simulink model "testRadiationDivisionInclined"  (R2018b)
settings: Solver=ode45  StartTime=0.0  StopTime=365*24*3600  MaxStep=100  RelTol=1e-3  EnableMultiTasking=on
undefined symbols (not defined in the file): Germany, path_carnot, Potsdam
libraries: carnot x3, Radiation_Divison x1
settings Model: Creator=drhf  LastModifiedBy=drhf
settings DataIOCC: LimitDataPoints=on  SaveFormat=Array  SignalLoggingSaveFormat=ModelDataLogs
settings OptimizationCC: ExpressionDepthLimit=2147483647  LifeSpan=inf
settings DebuggingCC: UnderspecifiedInitializationDetection=Classic  MergeDetectMultiDrivingBlocksExec=none  SolverPrmCheckMsg=warning  FcnCallInpInsideContextMsg=warning  StateNameClashWarn=warning  SFUnexpectedBacktrackingDiag=warning  SFNoUnconditionalDefaultTransitionDiag=warning  SFExecutionAtInitializationDiag=none
settings HardwareCC: ProdBitPerPointer=32  ProdBitPerSizeT=32  ProdBitPerPtrDiffT=32  ProdLargestAtomicFloat=None  ProdIntDivRoundTo=Undefined  ProdEndianess=Unspecified  ProdWordSize=32  ProdHWDeviceType=32-bit Generic
settings ModelReferenceCC: PropagateSignalLabelsOutOfModel=off
settings SFSimCC: SimUseLocalCustomCode=off
settings RTWCC: RTWUseLocalCustomCode=off
settings CodeAppCC: StateflowObjectComments=on
settings GRTTargetCC: TargetLangStandard=C89/C90 (ANSI)  GeneratePreprocessorConditionals=Disable all  CombineOutputUpdateFcns=off  GRTInterface=on
settings ConfigComp: CovMetricSettings=dw  CovHtmlReporting=on  CovSaveCumulativeToWorkspaceVar=on  CovSaveSingleToWorkspaceVar=on  CovExternalEMLEnable=off

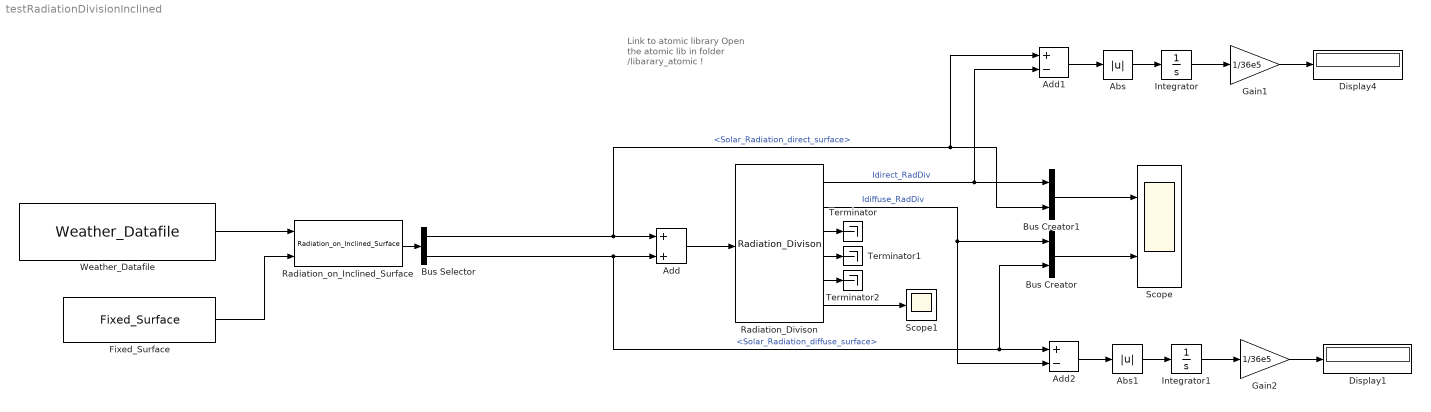
== system testRadiationDivisionInclined ==
  note: Link to atomic library
      | Open the atomic lib in
      | folder /libarary_atomic !
  Abs : Abs
  Abs1 : Abs
  Add : Sum
  Add1 : Sum  Inputs=+-
  Add2 : Sum  Inputs=+-
  Bus Creator : BusCreator  Inputs=2
  Bus Creator1 : BusCreator  Inputs=2
  Bus Selector : BusSelector  OutputSignals=Solar_Radiation_direct_surface,Solar_Radiation_diffuse_surface
  Display1 : Display
  Display4 : Display
  Fixed_Surface : carnot/Weather/Fixed_Surface  colangle=0  colazi=0  colrot=0
      settings: SourceProductName=Carnot
  Gain1 : Gain  Gain=1/36e5
  Gain2 : Gain  Gain=1/36e5
  Integrator : Integrator
  Integrator1 : Integrator
  Radiation_Divison : Radiation_Divison/Radiation_Divison  latitude=52.393800 % Potsdam / Germany  longitude=-13.065100 % Potsdam  longitude0="-15  % CET"
  Radiation_on_Inclined_Surface : carnot/Weather/Radiation_on_Inclined_Surface  sky=Perez 1990  reflect=0.2
      settings: SourceProductName=Carnot
  Scope : Scope  NumInputPorts=2
  Scope1 : Scope
  Terminator : Terminator
  Terminator1 : Terminator
  Terminator2 : Terminator
  Weather_Datafile : carnot/Weather/Weather_Datafile  PathName=path_carnot('data')  FileName='DE_TRY2016_Potsdam_averageYear.mat'  UserParam=off  VariableName=DE_TRY2010_04_averageYear  SampleTime=3600
      settings: SourceProductName=Carnot
  wires:
  Radiation_Divison/1 -> Add1/2, Bus Creator1/1  "Idirect_RadDiv"
  Radiation_Divison/2 -> Add2/2, Bus Creator/1  "Idiffuse_RadDiv"
  Radiation_Divison/3 -> Terminator/1
  Radiation_Divison/4 -> Terminator1/1
  Radiation_Divison/5 -> Terminator2/1
  Bus Selector/1 -> Add1/1, Bus Creator1/2, Add/1  "<Solar_Radiation_direct_surface>"
  Add/1 -> Radiation_Divison/1
  Bus Selector/2 -> Add2/1, Bus Creator/2, Add/2  "<Solar_Radiation_diffuse_surface>"
  Bus Creator1/1 -> Scope/1
  Bus Creator/1 -> Scope/2
  Add1/1 -> Abs/1
  Fixed_Surface/1 -> Radiation_on_Inclined_Surface/2
  Radiation_on_Inclined_Surface/1 -> Bus Selector/1
  Weather_Datafile/1 -> Radiation_on_Inclined_Surface/1
  Radiation_Divison/6 -> Scope1/1
  Abs/1 -> Integrator/1
  Integrator/1 -> Gain1/1
  Gain1/1 -> Display4/1
  Gain2/1 -> Display1/1
  Integrator1/1 -> Gain2/1
  Abs1/1 -> Integrator1/1
  Add2/1 -> Abs1/1
